simulink library "tpm"  (R2021b)
settings: Solver=VariableStepAuto  StartTime=0.0  StopTime=10.0  RelTol=1e-3
undefined symbols (not defined in the file or in its folder): ENUM_AN_LF, ENUM_AN_LR, ENUM_AN_RF, ENUM_AN_RR, ENUM_POWERSTA_OFF, ENUM_POWERSTA_OFFA, ENUM_POWERSTA_OFFC, ENUM_POWERSTA_ON, ENUM_POWERSTA_READY, ENUM_POWERSTA_STANDBY, ENUM_PWRSTASW_OFF, ENUM_PWRSTASW_OFFA, ENUM_PWRSTASW_OFFCHVCHRG, ENUM_PWRSTASW_STANDBY, ENUM_TPMSSNESORIDREGSTA_START, FALSE, KTPM_DataInVehSpdThreshold_kph, KTPM_Delay_raw8, KTPM_DiagLearn_flg, KTPM_TPMSModelVersion_raw, KTPM_TPMSModelVersionInit_raw, KTPM_WhlRotDir_enum_ovrdflg, KTPM_WhlRotDir_enum_ovrdval, TRUE, ZERO_FLOAT, ZERO_INT
libraries: simulink x58, $bdroot x27, hcu_lib x24
(part 3 of 9)

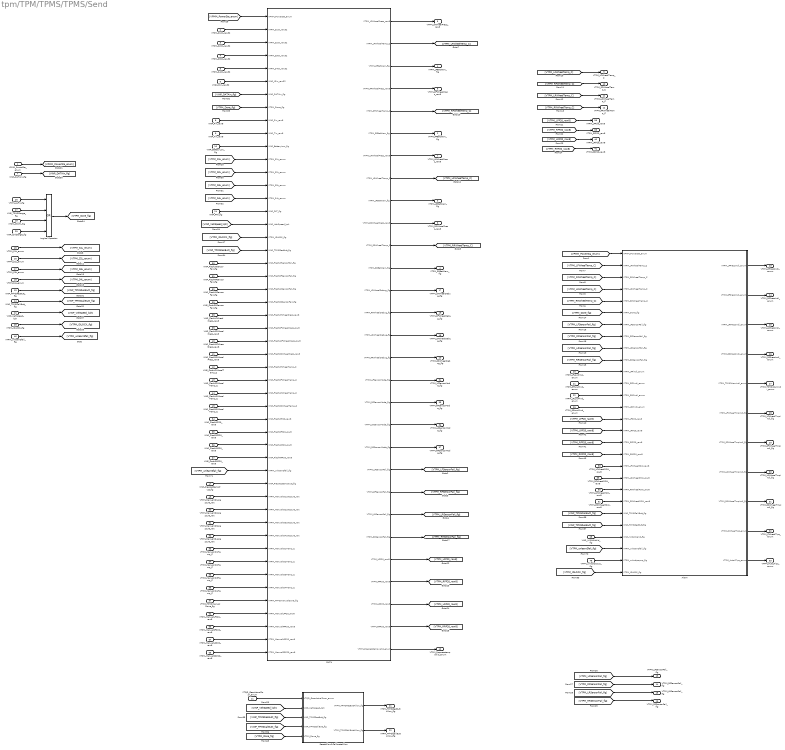
== system tpm/TPM/TPMS/TPMS/Send ==
  VPMM_PowerSta_enum : Inport
  VTPM_S1ID_raw32 : Inport  Port=2
  VTPM_S2ID_raw32 : Inport  Port=3
  VTPM_S3ID_raw32 : Inport  Port=4
  VTPM_S4ID_raw32 : Inport  Port=5
  VINP_IDin_raw32 : Inport  Port=6
  VINP_DATAin_flg : Inport  Port=7
  VINP_Pin_raw8 : Inport  Port=8
  VINP_Tin_raw8 : Inport  Port=9
  VINP_BatteryLow_flg : Inport  Port=10
  VTQD_GearActualPosn_enum : Inport  Port=11
  VINP_VehSpeed_kph : Inport  Port=12
  VINP_TPMSResButt_flg : Inport  Port=13
  VINP_TPMSCaliButt_flg : Inport  Port=14
  VTPM_S1L_enum : Inport  Port=15
  VTPM_S2L_enum : Inport  Port=16
  VTPM_S3L_enum : Inport  Port=17
  VTPM_S4L_enum : Inport  Port=18
  VTPM_Chkfin_flg : Inport  Port=19
  VTPM_LFLowPind_enum : Inport  Port=20
  VTPM_RFLowPind_enum : Inport  Port=21
  VTPM_LRLowPind_enum : Inport  Port=22
  VTPM_RRLowPind_enum : Inport  Port=23
  VINP_FAT_flg : Inport  Port=24
  VINP_IVICANValid_flg : Inport  Port=25
  VTPM_ALFin_flg : Inport  Port=26
  VINP_TPMSStorge_flg : Inport  Port=27
  VTPM_IDLOCK_flg : Inport  Port=28
  VINP_ChkStorge_flg : Inport  Port=29
  VINP_FlashLFSensorFail_flg : Inport  Port=30
  VINP_FlashRFSensorFail_flg : Inport  Port=31
  VINP_FlashLRSensorFail_flg : Inport  Port=32
  VINP_FlashRRSensorFail_flg : Inport  Port=33
  VINP_FlashLFP20_raw8 : Inport  Port=34
  VINP_FlashRFP20_raw8 : Inport  Port=35
  VINP_FlashLRP20_raw8 : Inport  Port=36
  VINP_FlashRRP20_raw8 : Inport  Port=37
  VINP_FlashLFWheelPress_raw8 : Inport  Port=38
  VINP_FlashRFWheelPress_raw8 : Inport  Port=39
  VINP_FlashLRFWheelPress_raw8 : Inport  Port=40
  VINP_FlashRRWheelPress_raw8 : Inport  Port=41
  VINP_FlashLFWheelTemp_C : Inport  Port=42
  VINP_FlashRFWheelTemp_C : Inport  Port=43
  VINP_FlashLRWheelTemp_C : Inport  Port=44
  VINP_FlashRRWheelTemp_C : Inport  Port=45
  VTPM_unlearnSfali_flg : Inport  Port=46
  VINP_Prepresstemptrust_flg : Inport  Port=47
  VTPM_unlockpopup_flg : Inport  Port=48
  VTPM_ManualID1pressure_raw : Inport  Port=49
  VTPM_ManualID2pressure_raw : Inport  Port=50
  VTPM_ManualID3pressure_raw : Inport  Port=51
  VTPM_ManualID4pressure_raw : Inport  Port=52
  VTPM_ManualID1Temp_C : Inport  Port=53
  VTPM_ManualID2Temp_C : Inport  Port=54
  VTPM_ManualID3Temp_C : Inport  Port=55
  VTPM_ManualID4Temp_C : Inport  Port=56
  VTPM_TPMSmanualDone_flg : Inport  Port=57
  VTPM_LFWheelPSW_raw8 : Inport  Port=58
  VTPM_RFWheelPSW_raw8 : Inport  Port=59
  VTPM_LRWheelPSW_raw8 : Inport  Port=60
  VTPM_RRWheelPSW_raw8 : Inport  Port=61
  VTPM_ManualLFP20_raw8 : Inport  Port=62
  VTPM_ManualRFP20_raw8 : Inport  Port=63
  VTPM_ManualLRP20_raw8 : Inport  Port=64
  VTPM_ManualRRP20_raw8 : Inport  Port=65
  Alarm : Subsystem
  DATA : Subsystem
  Logical Operator : Logic  Operator=OR  Inputs=4  AllPortsSameDT=off  OutDataTypeStr=boolean
  ResetAllow&CalibrateAllow : Subsystem
  "VTPM_LFBatWarn_flg " : Outport
  "VTPM_RFBatWarn_flg " : Outport  Port=2
  "VTPM_LRBatWarn_flg " : Outport  Port=3
  VTPM_RRBatWarn_flg : Outport  Port=4
  VTPM_LFWheelPress_raw8 : Outport  Port=5
  VTPM_RFWheelPress_raw8 : Outport  Port=6
  VTPM_LRWheelPress_raw8 : Outport  Port=7
  VTPM_RRWheelPress_raw8 : Outport  Port=8
  VTPM_LFWheelTemp_C : Outport  Port=9
  VTPM_RFWheelTemp_C : Outport  Port=10
  VTPM_LRWheelTemp_C : Outport  Port=11
  VTPM_RRWheelTemp_C : Outport  Port=12
  VTPM_LFSensorFail_flg : Outport  Port=13
  VTPM_RFSensorFail_flg : Outport  Port=14
  VTPM_LRSensorFail_flg : Outport  Port=15
  VTPM_RRSensorFail_flg : Outport  Port=16
  VTPM_LFWheelDebug_flg : Outport  Port=17
  VTPM_LRWheelDebug_flg : Outport  Port=18
  VTPM_RFWheelDebug_flg : Outport  Port=19
  VTPM_RRWheelDebug_flg : Outport  Port=20
  VTPM_TPMSResButtAllow_flg : Outport  Port=21
  VTPM_TPMSCaliButtAllow_flg : Outport  Port=22
  VTPM_LFPressIndi_enum : Outport  Port=23
  VTPM_RFPressIndi_enum : Outport  Port=24
  VTPM_LRPressIndi_enum : Outport  Port=25
  VTPM_RRPressIndi_enum : Outport  Port=26
  "VTPM_TPMSWarnIndi_enum " : Outport  Port=27
  VTPM_LFWheelTmpIndi_flg : Outport  Port=28
  VTPM_RFWheelTmpIndi_flg : Outport  Port=29
  VTPM_LRWheelTmpIndi_flg : Outport  Port=30
  VTPM_RRWheelTmpIndi_flg : Outport  Port=31
  VTPM_CWheelTips_enum : Outport  Port=32
  VTPM_AutoLTips_enum : Outport  Port=33
  VTPM_LFSensorMode_flg : Outport  Port=34
  VTPM_RFSensorMode_flg : Outport  Port=35
  VTPM_LRSensorMode_flg : Outport  Port=36
  VTPM_RRSensorMode_flg : Outport  Port=37
  VTPM_LFP20_raw8 : Outport  Port=38
  VTPM_RFP20_raw8 : Outport  Port=39
  VTPM_LRP20_raw8 : Outport  Port=40
  VTPM_RRP20_raw8 : Outport  Port=41
  VTPM_Prepresstempvalid_enum : Outport  Port=42
  wires:
  VINP_VehSpeed_kph/1 -> [VINP_VehSpeed_kph]
  [VINP_VehSpeed_kph] -> ResetAllow&CalibrateAllow/2(VINP_VehSpeed_kph)
  Alarm/11(VTPM_AutoLTips_enum) -> VTPM_AutoLTips_enum/1
  Alarm/10(VTPM_CWheelTips_enum) -> VTPM_CWheelTips_enum/1
  [VINP_TPMSCaliButt_flg] -> ResetAllow&CalibrateAllow/4(VINP_TPMSCaliButt_flg)
  [VINP_TPMSResButt_flg] -> ResetAllow&CalibrateAllow/3(VINP_TPMSResButt_flg)
  VINP_TPMSCaliButt_flg/1 -> [VINP_TPMSCaliButt_flg]
  VINP_TPMSResButt_flg/1 -> [VINP_TPMSResButt_flg]
  [VTPM_Done_flg] -> ResetAllow&CalibrateAllow/5(VTPM_Done_flg)
  VINP_DATAin_flg/1 -> [VINP_DATAin_flg]
  VTPM_S4L_enum/1 -> [VTPM_S4L_enum]
  VTPM_S3L_enum/1 -> [VTPM_S3L_enum]
  VTPM_S2L_enum/1 -> [VTPM_S2L_enum]
  VTPM_S1L_enum/1 -> [VTPM_S1L_enum]
  Alarm/9(VTPM_RRWheelTmpIndi_flg) -> VTPM_RRWheelTmpIndi_flg/1
  Alarm/8(VTPM_LRWheelTmpIndi_flg) -> VTPM_LRWheelTmpIndi_flg/1
  Alarm/7(VTPM_RFWheelTmpIndi_flg) -> VTPM_RFWheelTmpIndi_flg/1
  Alarm/6(VTPM_LFWheelTmpIndi_flg) -> VTPM_LFWheelTmpIndi_flg/1
  Alarm/5("VTPM_TPMSWarnIndi_enum ") -> "VTPM_TPMSWarnIndi_enum "/1
  Alarm/4(VTPM_RRPressIndi_enum) -> VTPM_RRPressIndi_enum/1
  Alarm/3(VTPM_LRPressIndi_enum) -> VTPM_LRPressIndi_enum/1
  Alarm/2(VTPM_RFPressIndi_enum) -> VTPM_RFPressIndi_enum/1
  Alarm/1(VTPM_LFPressIndi_enum) -> VTPM_LFPressIndi_enum/1
  ResetAllow&CalibrateAllow/1(VTPM_TPMSResButtAllow_flg) -> VTPM_TPMSResButtAllow_flg/1
  VTQD_GearActualPosn_enum/1 -> ResetAllow&CalibrateAllow/1(VTQD_GearActualPosn_enum)
  [VTPM_LFSensorFail_flg] -> VTPM_LFSensorFail_flg/1
  [VTPM_LRSensorFail_flg] -> VTPM_LRSensorFail_flg/1
  VPMM_PowerSta_enum/1 -> [VPMM_PowerSta_enum]
  [VTPM_RRSensorFail_flg] -> VTPM_RRSensorFail_flg/1
  [VTPM_RFSensorFail_flg] -> VTPM_RFSensorFail_flg/1
  ResetAllow&CalibrateAllow/2(VTPM_TPMSCaliButtAllow_flg) -> VTPM_TPMSCaliButtAllow_flg/1
  [VPMM_PowerSta_enum] -> Alarm/1(VPMM_PowerSta_enum)
  [VTPM_LFWheelTemp_C] -> Alarm/2(VTPM_LFWheelTemp_C)
  [VTPM_RFWheelTemp_C] -> Alarm/3(VTPM_RFWheelTemp_C)
  [VTPM_RRWheelTemp_C] -> Alarm/5(VTPM_RRWheelTemp_C)
  [VTPM_LRWheelTemp_C] -> Alarm/4(VTPM_LRWheelTemp_C)
  [VTPM_Done_flg] -> Alarm/6(VTPM_Done_flg)
  [VTPM_LFSensorFail_flg] -> Alarm/7(VTPM_LFSensorFail_flg)
  [VTPM_RFSensorFail_flg] -> Alarm/8(VTPM_RFSensorFail_flg)
  [VTPM_LRSensorFail_flg] -> Alarm/9(VTPM_LRSensorFail_flg)
  [VTPM_RRSensorFail_flg] -> Alarm/10(VTPM_RRSensorFail_flg)
  [VTPM_LFP20_raw8] -> Alarm/15(VTPM_LFP20_raw8)
  [VTPM_LRP20_raw8] -> Alarm/16(VTPM_LRP20_raw8)
  [VTPM_RFP20_raw8] -> Alarm/17(VTPM_RFP20_raw8)
  [VTPM_RRP20_raw8] -> Alarm/18(VTPM_RRP20_raw8)
  VTPM_LFWheelPSW_raw8/1 -> Alarm/19(VTPM_LFWheelPSW_raw8)
  VTPM_RFWheelPSW_raw8/1 -> Alarm/20(VTPM_LRWheelPSW_raw8)
  VTPM_LRWheelPSW_raw8/1 -> Alarm/21(VTPM_RFWheelPSW_raw8)
  VTPM_RRWheelPSW_raw8/1 -> Alarm/22(VTPM_RRWheelPSW_raw8)
  [VINP_TPMSCaliButt_flg] -> Alarm/23(VINP_TPMSCaliButt_flg)
  [VINP_TPMSResButt_flg] -> Alarm/24(VINP_TPMSResButt_flg)
  VINP_IVICANValid_flg/1 -> Alarm/25(VINP_IVICANValid_flg)
  VTPM_IDLOCK_flg/1 -> [VTPM_IDLOCK_flg]
  VTPM_ALFin_flg/1 -> Logical Operator/1
  VINP_TPMSStorge_flg/1 -> Logical Operator/2
  VTPM_Chkfin_flg/1 -> Logical Operator/3
  VINP_ChkStorge_flg/1 -> Logical Operator/4
  Logical Operator/1 -> [VTPM_Done_flg]
  VTPM_unlearnSfali_flg/1 -> [VTPM_unlearnSfali_flg]
  [VTPM_unlearnSfali_flg] -> Alarm/26(VTPM_unlearnSfali_flg)
  DATA/1(VTPM_LFWheelPress_raw8) -> VTPM_LFWheelPress_raw8/1
  DATA/2(VTPM_LFWheelTemp_C) -> [VTPM_LFWheelTemp_C]
  DATA/3(VTPM_LFBatWarn_flg) -> "VTPM_LFBatWarn_flg "/1
  DATA/4(VTPM_RFWheelPress_raw8) -> VTPM_RFWheelPress_raw8/1
  DATA/5(VTPM_RFWheelTemp_C) -> [VTPM_RFWheelTemp_C]
  DATA/6(VTPM_RFBatWarn_flg) -> "VTPM_RFBatWarn_flg "/1
  DATA/7(VTPM_LRWheelPress_raw8) -> VTPM_LRWheelPress_raw8/1
  DATA/8(VTPM_LRWheelTemp_C) -> [VTPM_LRWheelTemp_C]
  DATA/9(VTPM_LRBatWarn_flg) -> "VTPM_LRBatWarn_flg "/1
  DATA/10(VTPM_RRWheelPress_raw8) -> VTPM_RRWheelPress_raw8/1
  DATA/11(VTPM_RRWheelTemp_C) -> [VTPM_RRWheelTemp_C]
  DATA/12(VTPM_RRBatWarn_flg) -> VTPM_RRBatWarn_flg/1
  DATA/14(VTPM_RFWheelDebug_flg) -> VTPM_RFWheelDebug_flg/1
  DATA/13(VTPM_LFWheelDebug_flg) -> VTPM_LFWheelDebug_flg/1
  DATA/15(VTPM_LRWheelDebug_flg) -> VTPM_LRWheelDebug_flg/1
  DATA/16(VTPM_RRWheelDebug_flg) -> VTPM_RRWheelDebug_flg/1
  DATA/17(VTPM_LFSensorMode_flg) -> VTPM_LFSensorMode_flg/1
  DATA/18(VTPM_RFSensorMode_flg) -> VTPM_RFSensorMode_flg/1
  DATA/19(VTPM_LRSensorMode_flg) -> VTPM_LRSensorMode_flg/1
  DATA/20(VTPM_RRSensorMode_flg) -> VTPM_RRSensorMode_flg/1
  DATA/21(VTPM_LFSensorFail_flg) -> [VTPM_LFSensorFail_flg]
  DATA/22(VTPM_RFSensorFail_flg) -> [VTPM_RFSensorFail_flg]
  DATA/23(VTPM_LRSensorFail_flg) -> [VTPM_LRSensorFail_flg]
  DATA/24(VTPM_RRSensorFail_flg) -> [VTPM_RRSensorFail_flg]
  DATA/26(VTPM_RFP20_raw8) -> [VTPM_RFP20_raw8]
  DATA/25(VTPM_LFP20_raw8) -> [VTPM_LFP20_raw8]
  DATA/28(VTPM_RRP20_raw8) -> [VTPM_RRP20_raw8]
  DATA/27(VTPM_LRP20_raw8) -> [VTPM_LRP20_raw8]
  DATA/29(VTPM_Prepresstempvalid_enum) -> VTPM_Prepresstempvalid_enum/1
  [VPMM_PowerSta_enum] -> DATA/1(VPMM_PowerSta_enum)
  VTPM_S1ID_raw32/1 -> DATA/2(VTPM_S1ID_raw32)
  VTPM_S2ID_raw32/1 -> DATA/3(VTPM_S2ID_raw32)
  VTPM_S3ID_raw32/1 -> DATA/4(VTPM_S3ID_raw32)
  VTPM_S4ID_raw32/1 -> DATA/5(VTPM_S4ID_raw32)
  VINP_IDin_raw32/1 -> DATA/6(VINP_IDin_raw32)
  [VINP_DATAin_flg] -> DATA/7(VINP_DATAin_flg)
  [VTPM_Done_flg] -> DATA/8(VTPM_Done_flg)
  VINP_Pin_raw8/1 -> DATA/9(VINP_Pin_raw8)
  VINP_Tin_raw8/1 -> DATA/10(VINP_Tin_raw8)
  VINP_BatteryLow_flg/1 -> DATA/11(VINP_BatteryLow_flg)
  [VTPM_S1L_enum] -> DATA/12(VTPM_S1L_enum)
  [VTPM_S2L_enum] -> DATA/13(VTPM_S2L_enum)
  [VTPM_S3L_enum] -> DATA/14(VTPM_S3L_enum)
  [VTPM_S4L_enum] -> DATA/15(VTPM_S4L_enum)
  [VINP_VehSpeed_kph] -> DATA/17(VINP_VehSpeed_kph)
  VINP_FAT_flg/1 -> DATA/16(VINP_FAT_flg)
  [VTPM_IDLOCK_flg] -> DATA/18(VTPM_IDLOCK_flg)
  [VINP_TPMSResButt_flg] -> DATA/19(VINP_TPMSResButt_flg)
  VINP_FlashLFSensorFail_flg/1 -> DATA/20(VINP_FlashLFSensorFail_flg)
  VINP_FlashRFSensorFail_flg/1 -> DATA/21(VINP_FlashRFSensorFail_flg)
  VINP_FlashLRSensorFail_flg/1 -> DATA/22(VINP_FlashLRSensorFail_flg)
  VINP_FlashRRSensorFail_flg/1 -> DATA/23(VINP_FlashRRSensorFail_flg)
  VINP_FlashLFWheelPress_raw8/1 -> DATA/24(VINP_FlashLFWheelPress_raw8)
  VINP_FlashRFWheelPress_raw8/1 -> DATA/25(VINP_FlashRFWheelPress_raw8)
  VINP_FlashLRFWheelPress_raw8/1 -> DATA/26(VINP_FlashLRFWheelPress_raw8)
  VINP_FlashRRWheelPress_raw8/1 -> DATA/27(VINP_FlashRRWheelPress_raw8)
  VINP_FlashLFWheelTemp_C/1 -> DATA/28(VINP_FlashLFWheelTemp_C)
  VINP_FlashRFWheelTemp_C/1 -> DATA/29(VINP_FlashRFWheelTemp_C)
  VINP_FlashLRWheelTemp_C/1 -> DATA/30(VINP_FlashLRWheelTemp_C)
  VINP_FlashRRWheelTemp_C/1 -> DATA/31(VINP_FlashRRWheelTemp_C)
  VINP_FlashLFP20_raw8/1 -> DATA/32(VINP_FlashLFP20_raw8)
  VINP_FlashRFP20_raw8/1 -> DATA/33(VINP_FlashRFP20_raw8)
  VINP_FlashLRP20_raw8/1 -> DATA/34(VINP_FlashLRP20_raw8)
  VINP_FlashRRP20_raw8/1 -> DATA/35(VINP_FlashRRP20_raw8)
  [VTPM_unlearnSfali_flg] -> DATA/36(VTPM_unlearnSfali_flg)
  [VTPM_LFWheelTemp_C] -> VTPM_LFWheelTemp_C/1
  [VTPM_RFWheelTemp_C] -> VTPM_RFWheelTemp_C/1
  [VTPM_LRWheelTemp_C] -> VTPM_LRWheelTemp_C/1
  [VTPM_RRWheelTemp_C] -> VTPM_RRWheelTemp_C/1
  [VTPM_LFP20_raw8] -> VTPM_LFP20_raw8/1
  [VTPM_RFP20_raw8] -> VTPM_RFP20_raw8/1
  [VTPM_LRP20_raw8] -> VTPM_LRP20_raw8/1
  [VTPM_RRP20_raw8] -> VTPM_RRP20_raw8/1
  VINP_Prepresstemptrust_flg/1 -> DATA/37(VINP_Prepresstemptrust_flg)
  VTPM_unlockpopup_flg/1 -> Alarm/27(VTPM_unlockpopup_flg)
  [VTPM_IDLOCK_flg] -> Alarm/28(VTPM_IDLOCK_flg)
  VTPM_ManualID1pressure_raw/1 -> DATA/38(VTPM_ManualID1pressure_raw)
  VTPM_ManualID2pressure_raw/1 -> DATA/39(VTPM_ManualID2pressure_raw)
  VTPM_ManualID3pressure_raw/1 -> DATA/40(VTPM_ManualID3pressure_raw)
  VTPM_ManualID4pressure_raw/1 -> DATA/41(VTPM_ManualID4pressure_raw)
  VTPM_ManualID1Temp_C/1 -> DATA/42(VTPM_ManualID1Temp_C)
  VTPM_ManualID2Temp_C/1 -> DATA/43(VTPM_ManualID2Temp_C)
  VTPM_ManualID3Temp_C/1 -> DATA/44(VTPM_ManualID3Temp_C)
  VTPM_ManualID4Temp_C/1 -> DATA/45(VTPM_ManualID4Temp_C)
  VTPM_TPMSmanualDone_flg/1 -> DATA/46(VTPM_TPMSmanualDone_flg)
  VTPM_RRLowPind_enum/1 -> Alarm/14(VTPM_LRPindi_enum)
  VTPM_LRLowPind_enum/1 -> Alarm/13(VTPM_RRPindi_enum)
  VTPM_RFLowPind_enum/1 -> Alarm/12(VTPM_RFPindi_enum)
  VTPM_LFLowPind_enum/1 -> Alarm/11(VTPM_LFPindi_enum)
  VTPM_ManualLFP20_raw8/1 -> DATA/47(VTPM_ManualLFP20_raw8)
  VTPM_ManualRFP20_raw8/1 -> DATA/48(VTPM_ManualRFP20_raw8)
  VTPM_ManualLRP20_raw8/1 -> DATA/49(VTPM_ManualLRP20_raw8)
  VTPM_ManualRRP20_raw8/1 -> DATA/50(VTPM_ManualRRP20_raw8)

== system tpm/TPM/TPMS/TPMS/Subsystem ==
  VTPM_S1ID_raw32 : Inport
  VTPM_S2ID_raw32 : Inport  Port=2
  VTPM_S3ID_raw32 : Inport  Port=3
  VTPM_S4ID_raw32 : Inport  Port=4
  VTPM_S1L_enum : Inport  Port=5
  VTPM_S2L_enum : Inport  Port=6
  VTPM_S3L_enum : Inport  Port=7
  VTPM_S4L_enum : Inport  Port=8
  VTPM_ALFin_flg : Inport  Port=9
  VTPM_Chkfin_flg : Inport  Port=10
  VINP_TPMSStorge_flg : Inport  Port=11
  VINP_ChkStorge_flg : Inport  Port=12
  VINP_TPMSResButt_flg : Inport  Port=13
  VTPM_TPMSmanualDone_flg : Inport  Port=14
  Enable : EnablePort
  Chart : Stateflow chart  TreatAsAtomicUnit=on
  Data Type Conversion{,1..7} (8 alike) : DataTypeConversion  OutDataTypeStr=uint32
  Data Type Conversion8 : DataTypeConversion  OutDataTypeStr=uint8
  Data Type Conversion9 : DataTypeConversion  OutDataTypeStr=uint8
  Logical Operator : Logic  Operator=OR  Inputs=4  AllPortsSameDT=off  OutDataTypeStr=boolean
  Logical Operator1 : Logic  Operator=OR  Inputs=3  AllPortsSameDT=off  OutDataTypeStr=boolean
  Logical Operator2 : Logic  Operator=OR  Inputs=3  AllPortsSameDT=off  OutDataTypeStr=boolean
  MATLAB Function : MATLAB Function  TreatAsAtomicUnit=on
  VTPM_WriteChkLFID_raw : Outport
  VTPM_WriteChkRFID_raw : Outport  Port=2
  VTPM_WriteChkLRID_raw : Outport  Port=3
  VTPM_WriteChkRRID_raw : Outport  Port=4
  VTPM_WriteChkfinLFID_raw : Outport  Port=5
  VTPM_WriteChkfinRFID_raw : Outport  Port=6
  VTPM_WriteChkfinLRID_raw : Outport  Port=7
  VTPM_WriteChkfinRRID_raw : Outport  Port=8
  VTPM_Flashchkdatavalid_enum : Outport  Port=9
  VTPM_Flashdatavalid_enum : Outport  Port=10
  wires:
  [VINP_TPMSStorge_flg] -> Logical Operator1/2
  [VTPM_Chkfin_flg] -> Logical Operator1/1
  [VINP_ChkStorge_flg] -> Logical Operator2/2
  [VTPM_ALFin_flg] -> Logical Operator2/1
  [VINP_TPMSStorge_flg] -> Logical Operator/4
  [VTPM_Chkfin_flg] -> Logical Operator/3
  [VINP_ChkStorge_flg] -> Logical Operator/2
  [VTPM_ALFin_flg] -> Logical Operator/1
  VTPM_Chkfin_flg/1 -> [VTPM_Chkfin_flg]
  VINP_ChkStorge_flg/1 -> [VINP_ChkStorge_flg]
  VTPM_ALFin_flg/1 -> [VTPM_ALFin_flg]
  [VTPM_SetChkId_flg] -> Chart/7(VTPM_SetChkId_flg)
  [VTPM_WriteLRID_raw] -> Chart/3(VTPM_WriteLRID_raw)
  [VTPM_WriteRFID_raw] -> Chart/2(VTPM_WriteRFID_raw)
  [VTPM_WriteLFID_raw] -> Chart/1(VTPM_WriteLFID_raw)
  [VTPM_WriteRRID_raw] -> Chart/4(VTPM_WriteRRID_raw)
  VINP_TPMSResButt_flg/1 -> Chart/6(VINP_TPMSResButt_flg)
  Chart/8(VTPM_WriteChkfinRRID_raw) -> Data Type Conversion7/1
  Chart/5(VTPM_WriteChkfinLFID_raw) -> Data Type Conversion4/1
  Chart/4(VTPM_WriteChkRRID_raw) -> Data Type Conversion3/1
  Chart/1(VTPM_WriteChkLFID_raw) -> Data Type Conversion/1
  VTPM_S4L_enum/1 -> MATLAB Function/8(S4L)
  VTPM_S3L_enum/1 -> MATLAB Function/7(S3L)
  Logical Operator2/1 -> [VTPM_SetChkId_flg]
  Logical Operator1/1 -> [VTPM_CheckFin_flg]
  MATLAB Function/1(LFID) -> [VTPM_WriteLFID_raw]
  MATLAB Function/4(RRID) -> [VTPM_WriteRRID_raw]
  MATLAB Function/2(RFID) -> [VTPM_WriteRFID_raw]
  MATLAB Function/3(LRID) -> [VTPM_WriteLRID_raw]
  VINP_TPMSStorge_flg/1 -> [VINP_TPMSStorge_flg]
  Logical Operator/1 -> MATLAB Function/9(set)
  VTPM_S3ID_raw32/1 -> MATLAB Function/3(S3ID)
  VTPM_S1ID_raw32/1 -> MATLAB Function/1(S1ID)
  VTPM_S2ID_raw32/1 -> MATLAB Function/2(S2ID)
  VTPM_S4ID_raw32/1 -> MATLAB Function/4(S4ID)
  VTPM_S1L_enum/1 -> MATLAB Function/5(S1L)
  VTPM_S2L_enum/1 -> MATLAB Function/6(S2L)
  Chart/2(VTPM_WriteChkLRID_raw) -> Data Type Conversion1/1
  Chart/3(VTPM_WriteChkRFID_raw) -> Data Type Conversion2/1
  [VTPM_CheckFin_flg] -> Chart/5(VTPM_CheckFin_flg)
  Chart/6(VTPM_WriteChkfinLRID_raw) -> Data Type Conversion5/1
  Chart/7(VTPM_WriteChkfinRFID_raw) -> Data Type Conversion6/1
  Chart/9(VTPM_Flashchkdatavalid_flg) -> Data Type Conversion8/1
  Chart/10(VTPM_Flashdatavalid_flg) -> Data Type Conversion9/1
  Data Type Conversion/1 -> VTPM_WriteChkLFID_raw/1
  Data Type Conversion1/1 -> VTPM_WriteChkLRID_raw/1
  Data Type Conversion2/1 -> VTPM_WriteChkRFID_raw/1
  Data Type Conversion3/1 -> VTPM_WriteChkRRID_raw/1
  Data Type Conversion4/1 -> VTPM_WriteChkfinLFID_raw/1
  Data Type Conversion5/1 -> VTPM_WriteChkfinLRID_raw/1
  Data Type Conversion6/1 -> VTPM_WriteChkfinRFID_raw/1
  Data Type Conversion7/1 -> VTPM_WriteChkfinRRID_raw/1
  Data Type Conversion8/1 -> VTPM_Flashchkdatavalid_enum/1
  Data Type Conversion9/1 -> VTPM_Flashdatavalid_enum/1
  VTPM_TPMSmanualDone_flg/1 -> [VTPM_TPMSmanualDone_flg]
  [VTPM_TPMSmanualDone_flg] -> Logical Operator2/3
  [VTPM_TPMSmanualDone_flg] -> Logical Operator1/3

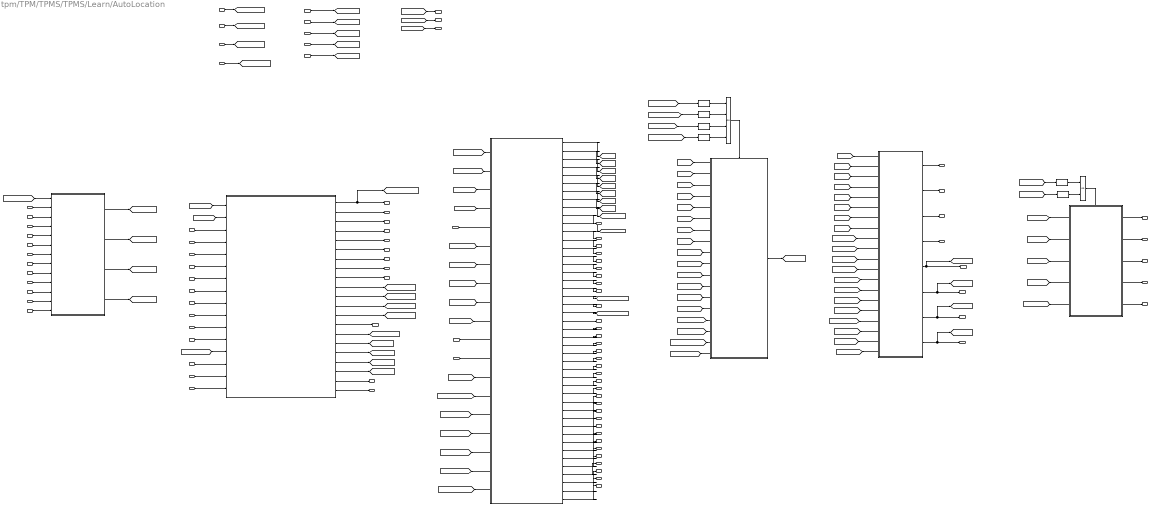
== system tpm/TPM/TPMS/TPMS/Learn/AutoLocation ==
  VINP_TPMSResButt_flg : Inport
  VINP_IDin_raw32 : Inport  Port=2
  VINP_DATAin_flg : Inport  Port=3
  VINP_FAT_flg : Inport  Port=4
  VPMM_PowerSta_enum : Inport  Port=5
  VINP_LFPulseCount_cnt : Inport  Port=6
  VINP_RFPulseCount_cnt : Inport  Port=7
  VINP_LRPulseCount_cnt : Inport  Port=8
  VINP_RRPulseCount_cnt : Inport  Port=9
  VINP_LFPulseCountV_flg : Inport  Port=10
  VINP_RFPulseCountV_flg : Inport  Port=11
  VINP_LRPulseCountV_flg : Inport  Port=12
  VINP_RRPulseCountV_flg : Inport  Port=13
  VTPM_LFWhlRotDir_enum : Inport  Port=14
  VTPM_RFWhlRotDir_enum : Inport  Port=15
  VTPM_LRWhlRotDir_enum : Inport  Port=16
  VTPM_RRWhlRotDir_enum : Inport  Port=17
  VINP_TPMSStorge_flg : Inport  Port=18
  VINP_LFID_raw : Inport  Port=19
  VINP_RFID_raw : Inport  Port=20
  VINP_LRID_raw : Inport  Port=21
  VINP_RRID_raw : Inport  Port=22
  VINP_ChkStorge_flg : Inport  Port=23
  VINP_ChkLFID_raw : Inport  Port=24
  VINP_ChkRFID_raw : Inport  Port=25
  VINP_ChkLRID_raw : Inport  Port=26
  VINP_ChkRRID_raw : Inport  Port=27
  VINP_VehSpeed_kph : Inport  Port=28
  VINP_FlashunlearnSfali_flg : Inport  Port=29
  VINP_S1ID_raw : Inport  Port=30
  VINP_S2ID_raw : Inport  Port=31
  VINP_S3ID_raw : Inport  Port=32
  VINP_S4ID_raw : Inport  Port=33
  VINP_Pin_raw8 : Inport  Port=34
  VINP_Tin_raw8 : Inport  Port=35
  VINP_TPMSTrigger_flg : Inport  Port=36
  VTPM_DiagLearn_flg : Inport  Port=37
  Detect Increase{,1..5} (6 alike) : simulink/Logic and Bit Operations/Detect Increase  vinit=0.0  OutDataTypeStr=boolean
  Doublecheck : Subsystem
  IDIdentify : Subsystem
  IDtrans : Subsystem
  Logical Operator : Logic  Operator=OR  Inputs=4  AllPortsSameDT=off  OutDataTypeStr=boolean
  Logical Operator1 : Logic  Operator=OR  AllPortsSameDT=off  OutDataTypeStr=boolean
  Subsystem : Subsystem
  Subsystem1 : Subsystem
  WheelPosition : Subsystem
  VTPM_S1L_enum : Outport
  S1ID : Outport  Port=2
  VTPM_S2L_enum : Outport  Port=3
  S2ID : Outport  Port=4
  VTPM_S3L_enum : Outport  Port=5
  S3ID : Outport  Port=6
  VTPM_S4L_enum : Outport  Port=7
  S4ID : Outport  Port=8
  VTPM_LFS1_cnt : Outport  Port=9
  VTPM_RFS1_cnt : Outport  Port=10
  VTPM_RRS1_cnt : Outport  Port=11
  VTPM_LRS1_cnt : Outport  Port=12
  VTPM_LFS2_cnt : Outport  Port=13
  VTPM_RFS2_cnt : Outport  Port=14
  VTPM_RRS2_cnt : Outport  Port=15
  VTPM_LRS2_cnt : Outport  Port=16
  VTPM_LFS3_cnt : Outport  Port=17
  VTPM_RFS3_cnt : Outport  Port=18
  VTPM_RRS3_cnt : Outport  Port=19
  VTPM_LRS3_cnt : Outport  Port=20
  VTPM_LFS4_cnt : Outport  Port=21
  VTPM_RFS4_cnt : Outport  Port=22
  VTPM_RRS4_cnt : Outport  Port=23
  VTPM_LRS4_cnt : Outport  Port=24
  VTPM_IDLOCK_flg : Outport  Port=25
  VINP_FATAND_flg : Outport  Port=26
  VTPM_ALLFin_flg : Outport  Port=27
  VTPM_S1WheelDebugALTU_pct : Outport  Port=28
  VTPM_S2WheelDebugALTU_pct : Outport  Port=29
  VTPM_S3WheelDebugALTU_pct : Outport  Port=30
  VTPM_S4WheelDebugALTU_pct : Outport  Port=31
  VTPM_ID1messageALTU_raw8 : Outport  Port=32
  VTPM_ID2messageALTU_raw8 : Outport  Port=33
  VTPM_ID3messageALTU_raw8 : Outport  Port=34
  VTPM_ID4messageALTU_raw8 : Outport  Port=35
  VTPM_SetIDLoc_flg : Outport  Port=36
  VTPM_Chkfin_flg : Outport  Port=37
  VTPM_unlearnSfali_flg : Outport  Port=38
  VTPM_unlearnSfailvalid_enum : Outport  Port=39
  VTPM_FlashS1ID_raw : Outport  Port=40
  VTPM_FlashS2ID_raw : Outport  Port=41
  VTPM_FlashS3ID_raw : Outport  Port=42
  VTPM_FlashS4ID_raw : Outport  Port=43
  VTPM_FlashIDvalid_enum : Outport  Port=44
  VTPM_S1timeout_flg : Outport  Port=45
  VTPM_S2timeout_flg : Outport  Port=46
  VTPM_S3timeout_flg : Outport  Port=47
  VTPM_S4timeout_flg : Outport  Port=48
  VTPM_unlockpopup_flg : Outport  Port=49
  VTPM_ManualID1pressure_raw : Outport  Port=50
  VTPM_ManualID2pressure_raw : Outport  Port=51
  VTPM_ManualID3pressure_raw : Outport  Port=52
  VTPM_ManualID4pressure_raw : Outport  Port=53
  VTPM_ManualID1Temp_C : Outport  Port=54
  VTPM_ManualID2Temp_C : Outport  Port=55
  VTPM_ManualID3Temp_C : Outport  Port=56
  VTPM_ManualID4Temp_C : Outport  Port=57
  VTPM_TPMSmanualDone_flg : Outport  Port=58
  VTPM_WritingCnt_enum : Outport  Port=59
  VTPM_TPMSTLCmd_flg : Outport  Port=60
  VTPM_LProgress_enum : Outport  Port=61
  wires:
  WheelPosition/4(VTPM_LFWP_raw16) -> [VTPM_LFWP_raw16]  "VTPM_LFWP_raw16"
  WheelPosition/1(VTPM_RFWP_raw16) -> [VTPM_RFWP_raw16]  "VTPM_RFWP_raw16"
  VTPM_RFWhlRotDir_enum/1 -> WheelPosition/6(VTPM_RFWhlRotDir_enum)
  VINP_RRPulseCount_cnt/1 -> WheelPosition/13(VINP_RRPulseCount_cnt)
  VINP_LRPulseCount_cnt/1 -> WheelPosition/10(VINP_LRPulseCount_cnt)
  VINP_RFPulseCountV_flg/1 -> WheelPosition/5(VINP_RFPulseCountV_flg)
  VINP_LFPulseCountV_flg/1 -> WheelPosition/2(VINP_LFPulseCountV_flg)
  VINP_LFPulseCount_cnt/1 -> WheelPosition/4(VINP_LFPulseCount_cnt)
  VTPM_LFWhlRotDir_enum/1 -> WheelPosition/3(VTPM_LFWhlRotDir_enum)
  WheelPosition/2(VTPM_LRWP_raw16) -> [VTPM_LRWP_raw16]  "VTPM_LRWP_raw16"
  VTPM_LRWhlRotDir_enum/1 -> WheelPosition/9(VTPM_LRWhlRotDir_enum)
  VINP_RRPulseCountV_flg/1 -> WheelPosition/11(VINP_RRPulseCountV_flg)
  VINP_LRPulseCountV_flg/1 -> WheelPosition/8(VINP_LRPulseCountV_flg)
  VINP_RFPulseCount_cnt/1 -> WheelPosition/7(VINP_RFPulseCount_cnt)
  WheelPosition/3(VTPM_RRWP_raw16) -> [VTPM_RRWP_raw16]  "VTPM_RRWP_raw16"
  VTPM_RRWhlRotDir_enum/1 -> WheelPosition/12(VTPM_RRWhlRotDir_enum)
  VINP_DATAin_flg/1 -> [VINP_DATAin_flg]
  VINP_TPMSResButt_flg/1 -> [VINP_TPMSResButt_flg]
  VINP_IDin_raw32/1 -> [VINP_IDin_raw32]
  [S1L] -> IDtrans/1(S1L1)
  [S1ID] -> IDtrans/2(S1ID1)
  [S2L] -> IDtrans/3(S2L1)
  [S2ID] -> IDtrans/4(S2ID1)
  [S3L] -> IDtrans/5(S3L1)
  [S3ID] -> IDtrans/6(S3ID1)
  [S4L] -> IDtrans/7(S4L1)
  [S4ID] -> IDtrans/8(S4ID1)
  IDtrans/1(VTPM_S1L_enum) -> VTPM_S1L_enum/1
  IDtrans/5(S1ID) -> [VTPM_S1ID_raw], S1ID/1
  IDtrans/2(VTPM_S2L_enum) -> VTPM_S2L_enum/1
  IDtrans/6(S2ID) -> [VTPM_S2ID_raw], S2ID/1
  IDtrans/3(VTPM_S3L_enum) -> VTPM_S3L_enum/1
  IDtrans/7(S3ID) -> [VTPM_S3ID_raw], S3ID/1
  IDtrans/4(VTPM_S4L_enum) -> VTPM_S4L_enum/1
  IDtrans/8(S4ID) -> [VTPM_S4ID_raw], S4ID/1
  VPMM_PowerSta_enum/1 -> [VPMM_PowerSta_enum]
  [VPMM_PowerSta_enum] -> WheelPosition/1(VPMM_PowerSta_enum)
  VINP_ChkStorge_flg/1 -> [VINP_ChkStorge_flg]
  VINP_ChkLFID_raw/1 -> [VINP_ChkLFID_raw]
  VINP_ChkRFID_raw/1 -> [VINP_ChkRFID_raw]
  VINP_ChkLRID_raw/1 -> [VINP_ChkLRID_raw]
  VINP_ChkRRID_raw/1 -> [VINP_ChkRRID_raw]
  [VPMM_PowerSta_enum] -> IDIdentify/1(VPMM_PowerSta_enum)
  [VTPM_LFWP_raw16] -> IDIdentify/6(VTPM_LFWP_raw16)
  [VTPM_RFWP_raw16] -> IDIdentify/7(VTPM_RFWP_raw16)
  [VTPM_LRWP_raw16] -> IDIdentify/8(VTPM_LRWP_raw16)
  [VTPM_RRWP_raw16] -> IDIdentify/9(VTPM_RRWP_raw16)
  [VTPM_Chkfin_flg] -> IDIdentify/10(VTPM_Chkfin_flg)
  [VINP_TPMSResButt_flg] -> IDIdentify/2(VINP_TPMSResButt_flg)
  [VINP_IDin_raw32] -> IDIdentify/3(VINP_IDin_raw32)
  [VINP_DATAin_flg] -> IDIdentify/4(VINP_DATAin_flg)
  VINP_FAT_flg/1 -> IDIdentify/5(VINP_FAT_flg)
  Logical Operator/1 -> Doublecheck/Enable
  Detect Increase/1 -> Logical Operator/2
  [VINP_ChkRFID_raw] -> Doublecheck/12(VINP_ChkRFID_raw)
  [VTPM_DataEn] -> Detect Increase/1
  [VINP_TPMSResButt_flg] -> Detect Increase1/1
  Detect Increase1/1 -> Logical Operator/1
  [VINP_ChkRRID_raw] -> Doublecheck/14(VINP_ChkRRID_rawn5)
  [S3ID] -> Doublecheck/6(S3ID)
  [VINP_ChkStorge_flg] -> Doublecheck/10(VINP_ChkStorge_flg)
  Doublecheck/1(VTPM_Chkfin_flg) -> [VTPM_Chkfin_flg]
  [S2L] -> Doublecheck/3(S2L)
  [VINP_ChkLFID_raw] -> Doublecheck/11(VINP_ChkLFID_raw)
  [VTPM_Locdonetimes_cnt] -> Doublecheck/15(VTPM_Locdonetimes_cnt)
  [S4L] -> Doublecheck/7(S4L)
  [S3L] -> Doublecheck/5(S3L)
  [S1L] -> Doublecheck/1(S1L)
  [S1ID] -> Doublecheck/2(S1ID)
  [VINP_ChkLRID_raw] -> Doublecheck/13(VINP_ChkLRID_raw)
  [VTPM_ALLFin_flg] -> Doublecheck/9(VTPM_ALLFin_flg)
  [S2ID] -> Doublecheck/4(S2ID)
  [S4ID] -> Doublecheck/8(S4ID)
  IDIdentify/1(S1L) -> [S1L]
  IDIdentify/2(S1ID) -> [S1ID]
  IDIdentify/3(S2L) -> [S2L]
  IDIdentify/4(S2ID) -> [S2ID]
  IDIdentify/5(S3L) -> [S3L]
  IDIdentify/6(S3ID) -> [S3ID]
  IDIdentify/7(S4L) -> [S4L]
  IDIdentify/8(S4ID) -> [S4ID]
  IDIdentify/9(VTPM_IDLOCK_flg) -> [VTPM_IDLOCK_flg]
  IDIdentify/10(VINP_FATAND_flg) -> VINP_FATAND_flg/1
  IDIdentify/11(VTPM_ALLFIN_flg) -> [VTPM_ALLFin_flg]
  [VINP_ChkLFID_raw] -> IDtrans/13(VINP_ChkLFID_raw)
  [VINP_ChkRFID_raw] -> IDtrans/14(VINP_ChkRFID_raw)
  [VINP_ChkLRID_raw] -> IDtrans/15(VINP_ChkLRID_raw)
  [VINP_ChkRRID_raw] -> IDtrans/16(VINP_ChkRRID_raw)
  [VINP_ChkStorge_flg] -> IDtrans/18(VINP_ChkStorge_flg)
  [VTPM_ALLFin_flg] -> IDtrans/20(VTPM_ALLFin_flg)
  [VTPM_Chkfin_flg] -> IDtrans/19(VTPM_Chkfin_flg)
  VINP_VehSpeed_kph/1 -> IDIdentify/11(VINP_VehSpeed_kph)
  VINP_FlashunlearnSfali_flg/1 -> IDIdentify/12(VINP_FlashunlearnSfali_flg)
  [VTPM_ManuTPMSStorge_flg] -> IDtrans/17(VTPM_TPMSStorge_flg)
  [VINP_ChkStorge_flg] -> IDIdentify/13(VINP_ChkStorge_flg)
  [VTPM_ManuTPMSStorge_flg] -> IDIdentify/14(VINP_TPMSStorge_flg)
  Subsystem/5(VTPM_FlashIDvalid_enum) -> VTPM_FlashIDvalid_enum/1
  Subsystem/4(VTPM_FlashS4ID_raw) -> VTPM_FlashS4ID_raw/1
  Subsystem/3(VTPM_FlashS3ID_raw) -> VTPM_FlashS3ID_raw/1
  Subsystem/2(VTPM_FlashS2ID_raw) -> VTPM_FlashS2ID_raw/1
  Subsystem/1(VTPM_FlashS1ID_raw) -> VTPM_FlashS1ID_raw/1
  [VINP_TPMSResButt_flg] -> Subsystem/5(VINP_TPMSResButt_flg)
  Detect Increase3/1 -> Logical Operator1/2
  [VTPM_IDLOCK_flg] -> Detect Increase3/1
  Logical Operator1/1 -> Subsystem/Enable
  [VINP_TPMSResButt_flg] -> Detect Increase2/1
  Detect Increase2/1 -> Logical Operator1/1
  [VTPM_S4ID_raw] -> Subsystem/4(S4ID)
  [VTPM_S3ID_raw] -> Subsystem/3(S3ID)
  [VTPM_S2ID_raw] -> Subsystem/2(S2ID)
  [VTPM_S1ID_raw] -> Subsystem/1(S1ID)
  IDIdentify/12(VTPM_S1WheelDebugALTU_pct) -> VTPM_S1WheelDebugALTU_pct/1
  IDIdentify/13(VTPM_S2WheelDebugALTU_pct) -> VTPM_S2WheelDebugALTU_pct/1
  IDIdentify/14(VTPM_S3WheelDebugALTU_pct) -> VTPM_S3WheelDebugALTU_pct/1
  IDIdentify/15(VTPM_S4WheelDebugALTU_pct) -> VTPM_S4WheelDebugALTU_pct/1
  IDIdentify/16(VTPM_ID1messageALTU_raw8) -> VTPM_ID1messageALTU_raw8/1
  IDIdentify/17(VTPM_ID2messageALTU_raw8) -> VTPM_ID2messageALTU_raw8/1
  IDIdentify/18(VTPM_ID3messageALTU_raw8) -> VTPM_ID3messageALTU_raw8/1
  IDIdentify/19(VTPM_ID4messageALTU_raw8) -> VTPM_ID4messageALTU_raw8/1
  IDIdentify/20(VTPM_Locdonetimes_cnt) -> [VTPM_Locdonetimes_cnt]
  IDIdentify/21(VTPM_SetIDLoc_flg) -> VTPM_SetIDLoc_flg/1
  IDIdentify/22(VTPM_DataEn) -> [VTPM_DataEn]
  IDIdentify/40(VTPM_unlearnSfailvalid_enum) -> VTPM_unlearnSfailvalid_enum/1
  IDIdentify/23(VTPM_LFS1_cnt) -> VTPM_LFS1_cnt/1
  IDIdentify/24(VTPM_RFS1_cnt) -> VTPM_RFS1_cnt/1
  IDIdentify/25(VTPM_RRS1_cnt) -> VTPM_RRS1_cnt/1
  IDIdentify/26(VTPM_LRS1_cnt) -> VTPM_LRS1_cnt/1
  IDIdentify/27(VTPM_LFS2_cnt) -> VTPM_LFS2_cnt/1
  IDIdentify/28(VTPM_RFS2_cnt) -> VTPM_RFS2_cnt/1
  IDIdentify/29(VTPM_RRS2_cnt) -> VTPM_RRS2_cnt/1
  IDIdentify/30(VTPM_LRS2_cnt) -> VTPM_LRS2_cnt/1
  IDIdentify/31(VTPM_LFS3_cnt) -> VTPM_LFS3_cnt/1
  IDIdentify/32(VTPM_RFS3_cnt) -> VTPM_RFS3_cnt/1
  IDIdentify/33(VTPM_RRS3_cnt) -> VTPM_RRS3_cnt/1
  IDIdentify/34(VTPM_LRS3_cnt) -> VTPM_LRS3_cnt/1
  IDIdentify/35(VTPM_LFS4_cnt) -> VTPM_LFS4_cnt/1
  IDIdentify/36(VTPM_RFS4_cnt) -> VTPM_RFS4_cnt/1
  IDIdentify/37(VTPM_RRS4_cnt) -> VTPM_RRS4_cnt/1
  IDIdentify/38(VTPM_LRS4_cnt) -> VTPM_LRS4_cnt/1
  IDIdentify/39(VTPM_unlearnSfali_flg) -> VTPM_unlearnSfali_flg/1
  IDIdentify/43(VTPM_S3timeout_flg) -> VTPM_S3timeout_flg/1
  IDIdentify/44(VTPM_S4timeout_flg) -> VTPM_S4timeout_flg/1
  IDIdentify/41(VTPM_S1timeout_flg) -> VTPM_S1timeout_flg/1
  IDIdentify/42(VTPM_S2timeout_flg) -> VTPM_S2timeout_flg/1
  [VTPM_IDLOCK_flg] -> VTPM_IDLOCK_flg/1
  [VTPM_ALLFin_flg] -> VTPM_ALLFin_flg/1
  [VTPM_Chkfin_flg] -> VTPM_Chkfin_flg/1
  [VTPM_ManuTPMSStorge_flg] -> Doublecheck/16(VTPM_TPMSStorge_flg)
  [VTPM_ManuTPMSStorge_flg] -> Detect Increase4/1
  Detect Increase4/1 -> Logical Operator/3
  IDIdentify/45(VTPM_unlockpopup_flg) -> VTPM_unlockpopup_flg/1
  [VINP_IDin_raw32] -> Subsystem1/1(VINP_IDin_raw32)
  [VINP_DATAin_flg] -> Subsystem1/2(VINP_DATAin_flg)
  VINP_Pin_raw8/1 -> Subsystem1/3(VINP_Pin_raw8)
  VINP_Tin_raw8/1 -> Subsystem1/4(VINP_Tin_raw8)
  Subsystem1/1(VTPM_TPMSmanualDone_flg) -> [VTPM_TPMSmanualDone_flg], VTPM_TPMSmanualDone_flg/1
  [VTPM_TPMSmanualDone_flg] -> Detect Increase5/1
  Detect Increase5/1 -> Logical Operator/4
  [VTPM_TPMSmanualDone_flg] -> Doublecheck/17(VTPM_TPMSmanualDone_flg)
  Subsystem1/2(VTPM_ManualID1pressure_raw) -> VTPM_ManualID1pressure_raw/1
  Subsystem1/3(VTPM_ManualID2pressure_raw) -> VTPM_ManualID2pressure_raw/1
  Subsystem1/4(VTPM_ManualID3pressure_raw) -> VTPM_ManualID3pressure_raw/1
  Subsystem1/5(VTPM_ManualID4pressure_raw) -> VTPM_ManualID4pressure_raw/1
  Subsystem1/6(VTPM_ManualID1Temp_C) -> VTPM_ManualID1Temp_C/1
  Subsystem1/7(VTPM_ManualID2Temp_C) -> VTPM_ManualID2Temp_C/1
  Subsystem1/8(VTPM_ManualID3Temp_C) -> VTPM_ManualID3Temp_C/1
  Subsystem1/9(VTPM_ManualID4Temp_C) -> VTPM_ManualID4Temp_C/1
  [VTPM_TPMSmanualDone_flg] -> IDIdentify/19(VTPM_TPMSmanualDone_flg)
  VINP_S1ID_raw/1 -> Subsystem1/5(VINP_S1ID_raw)
  VINP_S2ID_raw/1 -> Subsystem1/6(VINP_S2ID_raw)
  VINP_S3ID_raw/1 -> Subsystem1/7(VINP_S3ID_raw)
  VINP_S4ID_raw/1 -> Subsystem1/8(VINP_S4ID_raw)
  Subsystem1/10(VTPM_MSensor1ID_raw) -> [VTPM_MSensor1ID_raw]
  Subsystem1/11(VTPM_MSensor2ID_raw) -> [VTPM_MSensor2ID_raw]
  Subsystem1/12(VTPM_MSensor3ID_raw) -> [VTPM_MSensor3ID_raw]
  Subsystem1/13(VTPM_MSensor4ID_raw) -> [VTPM_MSensor4ID_raw]
  [VTPM_MSensor1ID_raw] -> IDIdentify/15(VTPM_S1ID_raw)
  [VTPM_MSensor2ID_raw] -> IDIdentify/16(VTPM_S2ID_raw)
  [VTPM_MSensor3ID_raw] -> IDIdentify/17(VTPM_S3ID_raw)
  [VTPM_MSensor4ID_raw] -> IDIdentify/18(VTPM_S4ID_raw)
  [VINP_TPMSResButt_flg] -> Subsystem1/13(VINP_TPMSResButt_flg)
  [VINP_TPMSResButt_flg] -> Doublecheck/18(VINP_TPMSResButt_flg)
  Subsystem1/14(VTPM_WritingCnt_enum) -> VTPM_WritingCnt_enum/1
  Subsystem1/15(VTPM_ManuTPMSStorge_flg) -> [VTPM_ManuTPMSStorge_flg]
  [VTPM_MLFID_raw] -> IDtrans/9(VINP_LFID_raw)
  [VTPM_MRFID_raw] -> IDtrans/10(VINP_RFID_raw)
  [VTPM_MLRID_raw] -> IDtrans/11(VINP_LRID_raw)
  [VTPM_MRRID_raw] -> IDtrans/12(VINP_RRID_raw)
  VINP_LFID_raw/1 -> Subsystem1/9(VINP_LFID_raw)
  VINP_RFID_raw/1 -> Subsystem1/10(VINP_RFID_raw)
  VINP_LRID_raw/1 -> Subsystem1/11(VINP_LRID_raw)
  VINP_RRID_raw/1 -> Subsystem1/12(VINP_RRID_raw)
  Subsystem1/16(VTPM_MLFID_raw) -> [VTPM_MLFID_raw]
  Subsystem1/17(VTPM_MLRID_raw) -> [VTPM_MLRID_raw]
  Subsystem1/18(VTPM_MRFID_raw) -> [VTPM_MRFID_raw]
  Subsystem1/19(VTPM_MRRID_raw) -> [VTPM_MRRID_raw]
  VINP_TPMSStorge_flg/1 -> Subsystem1/14(VINP_TPMSStorge_flg)
  VINP_TPMSTrigger_flg/1 -> Subsystem1/15(VINP_TPMSTrigger_flg)
  Subsystem1/20(VTPM_TPMSTLCmd_flg) -> VTPM_TPMSTLCmd_flg/1
  VTPM_DiagLearn_flg/1 -> Subsystem1/16(VTPM_DiagLearn_flg)
  Subsystem1/21(VTPM_LProgress_enum) -> VTPM_LProgress_enum/1

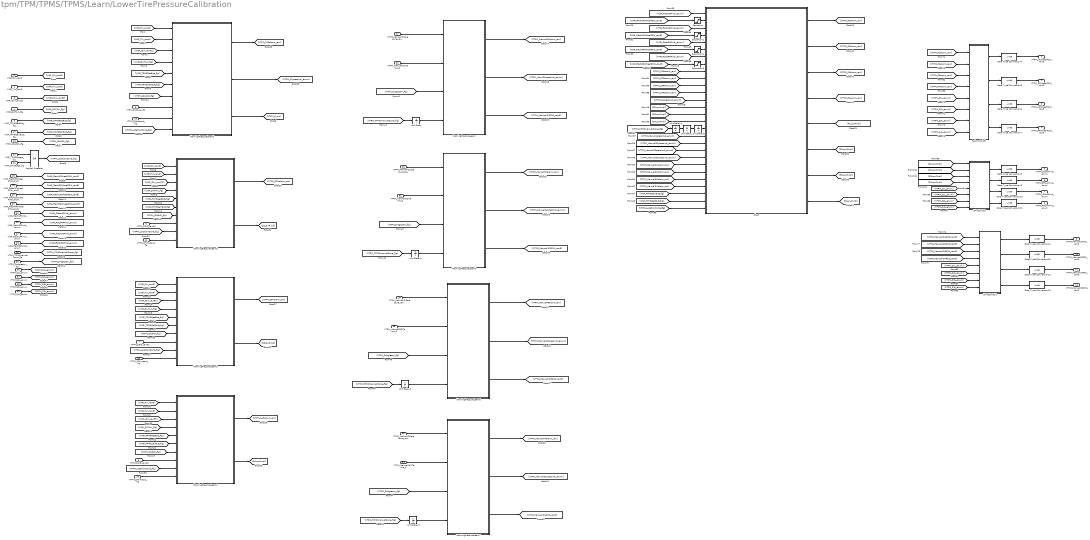
== system tpm/TPM/TPMS/TPMS/Learn/LowerTirePressureCalibration ==
  VINP_Pin_raw8 : Inport
  VINP_Tin_raw8 : Inport  Port=2
  VINP_IDin_raw32 : Inport  Port=3
  VINP_DATAin_flg : Inport  Port=4
  VTPM_S1ID_raw32 : Inport  Port=5
  VTPM_S2ID_raw32 : Inport  Port=6
  VTPM_S3ID_raw32 : Inport  Port=7
  VTPM_S4ID_raw32 : Inport  Port=8
  VINP_TPMSResButt_flg : Inport  Port=9
  VTPM_IDLOCK_flg : Inport  Port=10
  VINP_TPMSStorge_flg : Inport  Port=11
  VINP_ChkStorge_flg : Inport  Port=12
  VTPM_S1timeout_flg : Inport  Port=13
  VTPM_S2timeout_flg : Inport  Port=14
  VTPM_S4timeout_flg : Inport  Port=15
  VTPM_S3timeout_flg : Inport  Port=16
  VINP_TPMSCaliButt_flg : Inport  Port=17
  VINP_FlashLFWheelPSW_raw8 : Inport  Port=18
  VINP_FlashRFWheelPSW_raw8 : Inport  Port=19
  VINP_FlashLRWheelPSW_raw8 : Inport  Port=20
  VINP_FlashRRWheelPSW_raw8 : Inport  Port=21
  VINP_FlashLFPindi_enum : Inport  Port=22
  VINP_FlashRFPindi_enum : Inport  Port=23
  VINP_FlashLRPindi_enum : Inport  Port=24
  VINP_FlashRRPindi_enum : Inport  Port=25
  VTPM_TPMSmanualDone_flg : Inport  Port=26
  VTPM_ManualID1pressure_raw : Inport  Port=27
  VTPM_ManualID2pressure_raw : Inport  Port=28
  VTPM_ManualID3pressure_raw : Inport  Port=29
  VTPM_ManualID4pressure_raw : Inport  Port=30
  VTPM_ManualID1Temp_C : Inport  Port=31
  VTPM_ManualID2Temp_C : Inport  Port=32
  VTPM_ManualID3Temp_C : Inport  Port=33
  VTPM_ManualID4Temp_C : Inport  Port=34
  VTPM_DiagLearn_flg : Inport  Port=35
  VTPM_S1L_enum : Inport  Port=36
  VTPM_S2L_enum : Inport  Port=37
  VTPM_S3L_enum : Inport  Port=38
  VTPM_S4L_enum : Inport  Port=39
  Chart : Stateflow chart  TreatAsAtomicUnit=on
      settings: PortSchema="{\"entries\":[{\"content\":{\"sides\":[{\"content\":{\"connectorIds\":[\"In1\",\"In2\",\"In3\",\"In4\",\"In5\",\"In6\",\"In7\",\"In8\",\"In9\",\"In11\",\"In13\",\"In15\",\"In10\",\"In12\",\"In14\",\"In16\",\"In17\",\"In18\",\"In19\",\"In20\",\"In21\",\"In22\",\"In23\",\"In24\",\"In25\",\"In26\",\"In27\",\"In28\"]},\"type\":\"ConnectorPlacement.EquallySpacedRectSide\",\"uuid\":\"3e82d442-2b0d-4b76-abec-4e0dfebead9c\"},{\"content\":{\"connectorIds\":[\"Out1\",\"Out2\",\"Out3\",\"Out4\",\"Out5\",\"Out6\",\"Out7\",\"Out8\"],\"side\":\"RIGHT\"},\"type\":\"ConnectorPlacement.EquallySpacedRectSide\",\"uuid\":\"5058468e-7da9-4d60-9c1e-92187ef30700\"},{\"content\":{\"connectorIds\":[],\"side\":\"TOP\"},\"type\":\"ConnectorPlacement.EquallySpacedRectSide\",\"uuid\":\"68de6b22-e095-430f-837a-11b70d2d2994\"}]},\"type\":\"ConnectorPlacement.EquallySpacedConnector\",\"uuid\":\"48eb6e26-4b92-4f2c-bb39-a7d43f2c7c01\"}],\"packageUris\":[\"http://schema.mathworks.com/mf0/Connector/R2020b\"],\"version\":\"1.0\"}"
  Data Type Conversion{4..15} (12 alike) : DataTypeConversion  OutDataTypeStr=uint8
  LPindSwitch : MATLAB Function  TreatAsAtomicUnit=on
  LPindSwitch1 : MATLAB Function  TreatAsAtomicUnit=on
  Logical Operator : Logic  Operator=OR  AllPortsSameDT=off  OutDataTypeStr=boolean
  PalarmSwitch : MATLAB Function  TreatAsAtomicUnit=on
  Saturation{,1..3} (4 alike) : Saturate  UpperLimit=255  LowerLimit=93
  Unit Delay{,1..6} (7 alike) : UnitDelay  SampleTime=-1  HasFrameUpgradeWarning=on
  WarningPressureLearn : Stateflow chart  TreatAsAtomicUnit=on
  WarningPressureLearn1 : Stateflow chart  TreatAsAtomicUnit=on
  WarningPressureLearn2 : Stateflow chart  TreatAsAtomicUnit=on
  WarningPressureLearn3 : Stateflow chart  TreatAsAtomicUnit=on
  WarningPressureLearn4 : Stateflow chart  TreatAsAtomicUnit=on
  WarningPressureLearn5 : Stateflow chart  TreatAsAtomicUnit=on
  WarningPressureLearn6 : Stateflow chart  TreatAsAtomicUnit=on
  WarningPressureLearn7 : Stateflow chart  TreatAsAtomicUnit=on
  VTPM_LFWheelPSW_raw8 : Outport
  VTPM_RFWheelPSW_raw8 : Outport  Port=2
  VTPM_LRWheelPSW_raw8 : Outport  Port=3
  VTPM_RRWheelPSW_raw8 : Outport  Port=4
  VTPM_LFLowPind_enum : Outport  Port=5
  VTPM_RFLowPind_enum : Outport  Port=6
  VTPM_LRLowPind_enum : Outport  Port=7
  VTPM_RRLowPind_enum : Outport  Port=8
  VTPM_ManualLFP20_raw8 : Outport  Port=9
  VTPM_ManualRFP20_raw8 : Outport  Port=10
  VTPM_ManualLRP20_raw8 : Outport  Port=11
  VTPM_ManualRRP20_raw8 : Outport  Port=12
  wires:
  VINP_Pin_raw8/1 -> [VINP_Pin_raw8]
  VINP_Tin_raw8/1 -> [VINP_Tin_raw8]
  VINP_IDin_raw32/1 -> [VINP_IDin_raw32]
  VINP_DATAin_flg/1 -> [VINP_DATAin_flg]
  VINP_TPMSResButt_flg/1 -> [VINP_TPMSResButt_flg]
  VINP_TPMSCaliButt_flg/1 -> [VINP_TPMSCaliButt_flg]
  [VINP_Pin_raw8] -> WarningPressureLearn1/1(VINP_Pin_raw8)
  [VINP_Tin_raw8] -> WarningPressureLearn1/2(VINP_Tin_raw8)
  [VINP_IDin_raw32] -> WarningPressureLearn1/3(VINP_IDin_raw32)
  [VINP_DATAin_flg] -> WarningPressureLearn1/4(VINP_DATAin_flg)
  [VINP_TPMSResButt_flg] -> WarningPressureLearn1/5(VINP_TPMSResButt_flg)
  [VINP_TPMSCaliButt_flg] -> WarningPressureLearn1/6(VINP_TPMSCaliButt_flg)
  VTPM_S1ID_raw32/1 -> WarningPressureLearn1/8(VTPM_S1ID_raw32)
  [VINP_TPMSResButt_flg] -> WarningPressureLearn3/5(VINP_TPMSResButt_flg)
  [VINP_IDin_raw32] -> WarningPressureLearn3/3(VINP_IDin_raw32)
  [VINP_DATAin_flg] -> WarningPressureLearn3/4(VINP_DATAin_flg)
  [VINP_Pin_raw8] -> WarningPressureLearn3/1(VINP_Pin_raw8)
  [VINP_Tin_raw8] -> WarningPressureLearn3/2(VINP_Tin_raw8)
  [VINP_TPMSCaliButt_flg] -> WarningPressureLearn3/6(VINP_TPMSCaliButt_flg)
  [VINP_TPMSResButt_flg] -> WarningPressureLearn4/5(VINP_TPMSResButt_flg)
  [VINP_IDin_raw32] -> WarningPressureLearn4/3(VINP_IDin_raw32)
  [VINP_DATAin_flg] -> WarningPressureLearn4/4(VINP_DATAin_flg)
  [VINP_Pin_raw8] -> WarningPressureLearn4/1(VINP_Pin_raw8)
  [VINP_Tin_raw8] -> WarningPressureLearn4/2(VINP_Tin_raw8)
  [VINP_TPMSCaliButt_flg] -> WarningPressureLearn4/6(VINP_TPMSCaliButt_flg)
  WarningPressureLearn1/2(VTPM_S1pressindi_enum) -> [VTPM_S1pressindi_enum]  "VTPM_Spressindi_enum"
  WarningPressureLearn5/1(VTPM_P2alarm_raw) -> [VTPM_S2Palarm_raw]
  WarningPressureLearn5/2(SPressindi) -> [S2LowPindi]
  VTPM_S4ID_raw32/1 -> WarningPressureLearn4/8(VTPM_S4ID_raw32)
  VTPM_S3ID_raw32/1 -> WarningPressureLearn3/8(VTPM_S3ID_raw32)
  WarningPressureLearn3/2(SPressindi) -> [S3LowPindi]
  WarningPressureLearn4/2(SPressindi) -> [S4LowPindi]
  WarningPressureLearn1/3(C) -> [VTPM_C_cnt]  "VTPM_C_cnt"
  [VTPM_IDLOCK_flg] -> WarningPressureLearn1/7(VTPM_IDLOCK_flg)
  [VTPM_IDLOCK_flg] -> WarningPressureLearn3/7(VTPM_IDLOCK_flg)
  [VTPM_IDLOCK_flg] -> WarningPressureLearn4/7(VTPM_IDLOCK_flg)
  [VTPM_IDLOCK_flg] -> WarningPressureLearn5/7(VTPM_IDLOCK_flg)
  [VINP_TPMSResButt_flg] -> WarningPressureLearn5/5(VINP_TPMSResButt_flg)
  [VINP_TPMSCaliButt_flg] -> WarningPressureLearn5/6(VINP_TPMSCaliButt_flg)
  [VINP_IDin_raw32] -> WarningPressureLearn5/3(VINP_IDin_raw32)
  [VINP_DATAin_flg] -> WarningPressureLearn5/4(VINP_DATAin_flg)
  [VINP_Pin_raw8] -> WarningPressureLearn5/1(VINP_Pin_raw8)
  [VINP_Tin_raw8] -> WarningPressureLearn5/2(VINP_Tin_raw8)
  VTPM_S2ID_raw32/1 -> WarningPressureLearn5/8(VTPM_S2ID_raw32)
  VTPM_IDLOCK_flg/1 -> [VTPM_IDLOCK_flg]
  Logical Operator/1 -> [VTPM_LocationDone_flg]
  VINP_ChkStorge_flg/1 -> Logical Operator/2
  VINP_TPMSStorge_flg/1 -> Logical Operator/1
  VINP_FlashRFWheelPSW_raw8/1 -> [VINP_FlashRFWheelPSW_raw8]
  VINP_FlashLRWheelPSW_raw8/1 -> [VINP_FlashLRWheelPSW_raw8]
  VINP_FlashLFWheelPSW_raw8/1 -> [VINP_FlashLFWheelPSW_raw8]
  VINP_FlashRRWheelPSW_raw8/1 -> [VINP_FlashRRWheelPSW_raw8]
  VINP_FlashLFPindi_enum/1 -> [VINP_FlashLFPindi_enum]
  VINP_FlashRFPindi_enum/1 -> [VINP_FlashRFPindi_enum]
  VINP_FlashRRPindi_enum/1 -> [VINP_FlashRRPindi_enum]
  VINP_FlashLRPindi_enum/1 -> [VINP_FlashLRPindi_enum]
  [VTPM_LocationDone_flg] -> WarningPressureLearn5/9(VTPM_LocationDone_flg)
  [VTPM_LocationDone_flg] -> WarningPressureLearn3/9(VTPM_LocationDone_flg)
  [VTPM_LocationDone_flg] -> WarningPressureLearn4/9(VTPM_LocationDone_flg)
  VTPM_S1timeout_flg/1 -> WarningPressureLearn1/9(VTPM_S1timeout_flg)
  VTPM_S2timeout_flg/1 -> WarningPressureLearn5/10(VTPM_S2timeout_flg)
  VTPM_S3timeout_flg/1 -> WarningPressureLearn3/10(VTPM_S3timeout_flg)
  VTPM_S4timeout_flg/1 -> WarningPressureLearn4/10(VTPM_S4timeout_flg)
  [VTPM_DiagLearn_flg] -> WarningPressureLearn7/3(DiagLearn)
  WarningPressureLearn2/1(VTPM_P2alarm_raw) -> [VTPM_ManualP2alarm_raw]  "VTPM_ManualP2alarm_raw"
  WarningPressureLearn/2(VTPM_S1pressindi_enum) -> [VTPM_ManuS1pressindi_enum]  "VTPM_ManualS1pressindi_enum"
  WarningPressureLearn6/1(VTPM_P3alarm_raw) -> [VTPM_ManualP3alarm_raw]  "VTPM_ManualP3alarm_raw"
  [VTPM_DiagLearn_flg] -> WarningPressureLearn/3(DiagLearn)
  [VTPM_DiagLearn_flg] -> WarningPressureLearn2/3(DiagLearn)
  VTPM_ManualID1pressure_raw/1 -> WarningPressureLearn/1(VTPM_ManualID1pressure_raw)
  VTPM_ManualID1Temp_C/1 -> WarningPressureLearn/2(VTPM_ManualID1Temp_C)
  [VTPM_DiagLearn_flg] -> WarningPressureLearn6/3(DiagLearn)
  WarningPressureLearn6/2(VTPM_S3pressindi_enum) -> [VTPM_ManualS3pressindi_enum]  "VTPM_ManualS3pressindi_enum"
  WarningPressureLearn2/2(VTPM_S2pressindi_enum) -> [VTPM_ManualS2pressindi_enum]  "VTPM_ManualS2pressindi_enum"
  WarningPressureLearn7/2(VTPM_S4pressindi_enum) -> [VTPM_ManualS4pressindi_enum]  "VTPM_ManualS4pressindi_enum"
  WarningPressureLearn/1(VTPM_P1alarm_raw) -> [VTPM_ManualP1alarm_raw]  "VTPM_ManualP1alarm_raw"
  WarningPressureLearn7/1(VTPM_P4alarm_raw) -> [VTPM_ManualP4alarm_raw]  "VTPM_ManualP4alarm_raw"
  WarningPressureLearn1/1(VTPM_P1alarm_raw) -> [VTPM_S1Palarm_raw]
  WarningPressureLearn3/1(VTPM_P3alarm_raw) -> [VTPM_S3Palarm_raw]
  WarningPressureLearn4/1(VTPM_P4alarm_raw) -> [VTPM_S4Palarm_raw]
  VTPM_TPMSmanualDone_flg/1 -> [VTPM_TPMSmanualDone_flg]
  [VTPM_TPMSmanualDone_flg] -> Unit Delay/1
  Unit Delay/1 -> WarningPressureLearn/4(VTPM_TPMSmanualDone_flg)
  VTPM_ManualID2pressure_raw/1 -> WarningPressureLearn2/1(VTPM_ManualID2pressure_raw)
  VTPM_ManualID2Temp_C/1 -> WarningPressureLearn2/2(VTPM_ManualID2Temp_C)
  [VTPM_TPMSmanualDone_flg] -> Unit Delay1/1
  Unit Delay1/1 -> WarningPressureLearn2/4(VTPM_TPMSmanualDone_flg)
  Unit Delay2/1 -> WarningPressureLearn6/4(VTPM_TPMSmanualDone_flg)
  [VTPM_TPMSmanualDone_flg] -> Unit Delay2/1
  VTPM_ManualID3pressure_raw/1 -> WarningPressureLearn6/1(VTPM_ManualID3pressure_raw)
  VTPM_ManualID3Temp_C/1 -> WarningPressureLearn6/2(VTPM_ManualID3Temp_C)
  VTPM_ManualID4Temp_C/1 -> WarningPressureLearn7/2(VTPM_ManualID4Temp_C)
  VTPM_ManualID4pressure_raw/1 -> WarningPressureLearn7/1(VTPM_ManualID4pressure_raw)
  Unit Delay3/1 -> WarningPressureLearn7/4(VTPM_TPMSmanualDone_flg)
  [VTPM_TPMSmanualDone_flg] -> Unit Delay3/1
  VTPM_DiagLearn_flg/1 -> [VTPM_DiagLearn_flg]
  Data Type Conversion7/1 -> VTPM_RRWheelPSW_raw8/1
  [VTPM_S1L_enum] -> PalarmSwitch/5(S1L)
  Data Type Conversion6/1 -> VTPM_LRWheelPSW_raw8/1
  [VTPM_S2L_enum] -> PalarmSwitch/6(S2L)
  PalarmSwitch/1(LFP) -> Data Type Conversion4/1
  [VTPM_S3L_enum] -> PalarmSwitch/7(S3L)
  Data Type Conversion4/1 -> VTPM_LFWheelPSW_raw8/1
  PalarmSwitch/3(LRP) -> Data Type Conversion6/1
  PalarmSwitch/2(RFP) -> Data Type Conversion5/1
  [VTPM_S4L_enum] -> PalarmSwitch/8(S4L)
  Data Type Conversion5/1 -> VTPM_RFWheelPSW_raw8/1
  PalarmSwitch/4(RRP) -> Data Type Conversion7/1
  [VTPM_P1alarm_raw] -> PalarmSwitch/1(P1)
  [VTPM_P2alarm_raw] -> PalarmSwitch/2(P2)
  [VTPM_P3alarm_raw] -> PalarmSwitch/3(P3)
  [VTPM_P4alarm_raw] -> PalarmSwitch/4(P4)
  VTPM_S2L_enum/1 -> [VTPM_S2L_enum]
  VTPM_S1L_enum/1 -> [VTPM_S1L_enum]
  VTPM_S3L_enum/1 -> [VTPM_S3L_enum]
  VTPM_S4L_enum/1 -> [VTPM_S4L_enum]
  Data Type Conversion10/1 -> VTPM_LRLowPind_enum/1
  Data Type Conversion9/1 -> VTPM_RFLowPind_enum/1
  [VTPM_S1L_enum] -> LPindSwitch/5(S1L)
  LPindSwitch/3(LRP) -> Data Type Conversion10/1
  LPindSwitch/4(RRP) -> Data Type Conversion11/1
  LPindSwitch/1(LFP) -> Data Type Conversion8/1
  LPindSwitch/2(RFP) -> Data Type Conversion9/1
  [P4LowPindi] -> LPindSwitch/4(P4)
  Data Type Conversion11/1 -> VTPM_RRLowPind_enum/1
  Data Type Conversion8/1 -> VTPM_LFLowPind_enum/1
  [VTPM_S2L_enum] -> LPindSwitch/6(S2L)
  [VTPM_S3L_enum] -> LPindSwitch/7(S3L)
  [P3LowPindi] -> LPindSwitch/3(P3)
  [P1LowPindi] -> LPindSwitch/1(P1)
  [VTPM_S4L_enum] -> LPindSwitch/8(S4L)
  [P2LowPindi] -> LPindSwitch/2(P2)
  [VTPM_LocationDone_flg] -> WarningPressureLearn1/10(VTPM_LocationDone_flg)
  WarningPressureLearn/3(VTPM_ManualID1P20_raw8) -> [VTPM_ManualID1P20_raw8]  "VTPM_ManualID1P20_raw8"
  WarningPressureLearn2/3(VTPM_ManualID2P20_raw8) -> [VTPM_ManualID2P20_raw8]  "VTPM_ManualID2P20_raw8"
  WarningPressureLearn6/3(VTPM_ManualID3P20_raw8) -> [VTPM_ManualID3P20_raw8]  "VTPM_ManualID3P20_raw8"
  WarningPressureLearn7/3(VTPM_ManualID4P20_raw8) -> [VTPM_ManualID4P20_raw8]  "VTPM_ManualID4P20_raw8"
  [VTPM_S3L_enum] -> LPindSwitch1/7(S3L)
  [VTPM_S4L_enum] -> LPindSwitch1/8(S4L)
  [VTPM_S2L_enum] -> LPindSwitch1/6(S2L)
  [VTPM_S1L_enum] -> LPindSwitch1/5(S1L)
  [VTPM_ManualID2P20_raw8] -> LPindSwitch1/2(P2)
  [VTPM_ManualID3P20_raw8] -> LPindSwitch1/3(P3)
  [VTPM_ManualID1P20_raw8] -> LPindSwitch1/1(P1)
  [VTPM_ManualID4P20_raw8] -> LPindSwitch1/4(P4)
  Data Type Conversion15/1 -> VTPM_ManualRFP20_raw8/1
  Data Type Conversion13/1 -> VTPM_ManualRRP20_raw8/1
  Data Type Conversion14/1 -> VTPM_ManualLFP20_raw8/1
  Data Type Conversion12/1 -> VTPM_ManualLRP20_raw8/1
  LPindSwitch1/2(RFP) -> Data Type Conversion15/1
  LPindSwitch1/1(LFP) -> Data Type Conversion14/1
  LPindSwitch1/3(LRP) -> Data Type Conversion12/1
  LPindSwitch1/4(RRP) -> Data Type Conversion13/1
  Saturation3/1 -> Chart/8(VINP_FlashRRWheelPSW_raw8)
  Saturation2/1 -> Chart/6(VINP_FlashRFWheelPSW_raw8)
  Saturation1/1 -> Chart/4(VINP_FlashLRWheelPSW_raw8)
  Saturation/1 -> Chart/2(VINP_FlashLFWheelPSW_raw8)
  Unit Delay5/1 -> Unit Delay6/1
  Unit Delay4/1 -> Unit Delay5/1
  Unit Delay6/1 -> Chart/17(VTPM_TPMSmanualDone_flg)
  [VTPM_TPMSmanualDone_flg] -> Unit Delay4/1
  [VTPM_LocationDone_flg] -> Chart/28(VTPM_LocationDone_flg)
  [VINP_TPMSCaliButt_flg] -> Chart/26(VINP_TPMSCaliButt_flg)
  [VINP_TPMSResButt_flg] -> Chart/27(VINP_TPMSResButt_flg)
  [VTPM_ManualP4alarm_raw] -> Chart/25(VTPM_ManualP4alarm_raw)
  [VTPM_ManualP3alarm_raw] -> Chart/24(VTPM_ManualP3alarm_raw)
  [VTPM_ManualP2alarm_raw] -> Chart/23(VTPM_ManualP2alarm_raw)
  [VTPM_ManualP1alarm_raw] -> Chart/22(VTPM_ManualP1alarm_raw)
  [VTPM_ManualS4pressindi_enum] -> Chart/21(VTPM_ManuS4pressindi_enum)
  [VTPM_ManualS3pressindi_enum] -> Chart/20(VTPM_ManuS3pressindi_enum)
  [VTPM_ManualS2pressindi_enum] -> Chart/19(VTPM_ManuS2pressindi_enum)
  [VTPM_ManuS1pressindi_enum] -> Chart/18(VTPM_ManuS1pressindi_enum)
  [S4LowPindi] -> Chart/16(VTPM_S4pressindi_enum)
  [S3LowPindi] -> Chart/14(VTPM_S3pressindi_enum)
  [S2LowPindi] -> Chart/12(VTPM_S2pressindi_enum)
  [VTPM_S1pressindi_enum] -> Chart/10(VTPM_S1pressindi_enum)
  [VTPM_S4Palarm_raw] -> Chart/15(VTPM_S4Palarm_raw)
  [VTPM_S3Palarm_raw] -> Chart/13(VTPM_S3Palarm_raw)
  [VTPM_S2Palarm_raw] -> Chart/11(VTPM_S2Palarm_raw)
  [VTPM_S1Palarm_raw] -> Chart/9(VTPM_S1Palarm_raw)
  [VINP_FlashRRWheelPSW_raw8] -> Saturation3/1
  [VINP_FlashRRPindi_enum] -> Chart/7(VINP_FlashRRPindi_enum)
  [VINP_FlashRFPindi_enum] -> Chart/5(VINP_FlashRFPindi_enum)
  [VINP_FlashLRPindi_enum] -> Chart/3(VINP_FlashLRPindi_enum)
  [VINP_FlashLRWheelPSW_raw8] -> Saturation1/1
  [VINP_FlashRFWheelPSW_raw8] -> Saturation2/1
  [VINP_FlashLFPindi_enum] -> Chart/1(VINP_FlashLFPindi_enum)
  [VINP_FlashLFWheelPSW_raw8] -> Saturation/1
  Chart/8(VTPM_P4Pressindi_enum) -> [P4LowPindi]
  Chart/7(VTPM_P3Pressindi_enum) -> [P3LowPindi]
  Chart/6(VTPM_P2Pressindi_enum) -> [P2LowPindi]
  Chart/5(VTPM_P1Pressindi_enum) -> [P1LowPindi]
  Chart/4(VTPM_P4alarm_raw) -> [VTPM_P4alarm_raw]
  Chart/3(VTPM_P3alarm_raw) -> [VTPM_P3alarm_raw]
  Chart/2(VTPM_P2alarm_raw) -> [VTPM_P2alarm_raw]
  Chart/1(VTPM_P1alarm_raw) -> [VTPM_P1alarm_raw]
